simulink model "smm_with_grf_tilting_2d"  (R2014b)
settings: Solver=FixedStepDiscrete  StartTime=0.0  StopTime=inf  FixedStep=sample_time  RelTol=1e-3
undefined symbols (not defined in the file or in its folder): A_lpf_dtau, A_lpf_leg_spring, alpha_apex, alpha_max, alpha_min, B1_lpf_dtau, B1_lpf_leg_spring, B2_lpf_dtau, B2_lpf_leg_spring, boom_mount_angle, boom_pelvis_offset_angle, c_energy, contact_threshold, control_start_time, d_y_boom_com_offset, d_y_boom_hip_offset, d_y_com, desired_torso_angle, dx_avg_desired, enable_torso_wave, fcut_contact, ff_energy_l, ff_energy_r, g, g_reduced, h_boom, HIP_MTR_MAX_CONT_TORQUE, i_robot, initial_com_height, initial_dx, j_leg, j_motor, j_rotor, j_segments, k0_virtual, k_placement, k_sea, kd_lateral, kd_motor, kd_torso, kp_lateral, kp_motor, kp_raibert, kp_torso, l0_leg, l0_min_flight_time, l0_virtual, l0_virtual_raibert, l_boom_projected, l_max, l_retract_delta, l_retract_swing_max, l_retract_swing_min, l_seg, l_yaw_center_to_pelvis, lambda1, lambda2, lateral_offset, lateral_target_angle_left, lateral_target_angle_right ... (+40)
libraries: simulink x24, slrtlib x4, simulink_extras x2
(part 1 of 4)
settings Model: BufferReuse=off  Creator=wmartin  LastModifiedBy=wmartin
settings SolverCC: EnableConcurrentExecution=on
settings DataIOCC: MaxDataPoints=1000000000  SaveFormat=StructureWithTime
settings OptimizationCC: BlockReduction=off  OptimizeBlockIOStorage=off  BufferReuse=off  GlobalBufferReuse=off  ExpressionFolding=off  ExpressionDepthLimit=2147483647  LocalBlockOutputs=off  SimCompilerOptimization=On
settings DebuggingCC: UnderspecifiedInitializationDetection=Classic  MergeDetectMultiDrivingBlocksExec=none  StateNameClashWarn=warning
settings HardwareCC: ProdIntDivRoundTo=Zero  ProdEndianess=LittleEndian  ProdLongLongMode=on  ProdHWDeviceType=Generic->32-bit x86 compatible
settings ModelReferenceCC: UpdateModelReferenceTargets=IfOutOfDate  EnableParallelModelReferenceBuilds=on
settings RTWCC: SystemTargetFile=slrt.tlc  TemplateMakefile=slrt_default_tmf  Description=Simulink Real-Time  RTWVerbose=off  ProcessScript=slrt_make_rtw_hook  RTWCompilerOptimization=On
settings CodeAppCC: MaxIdLength=256
settings SimulinkRealTimeCC: GeneratePreprocessorConditionals=Disable all  EnableShiftOperators=on  RL32LogBufSizeModifier=100000000

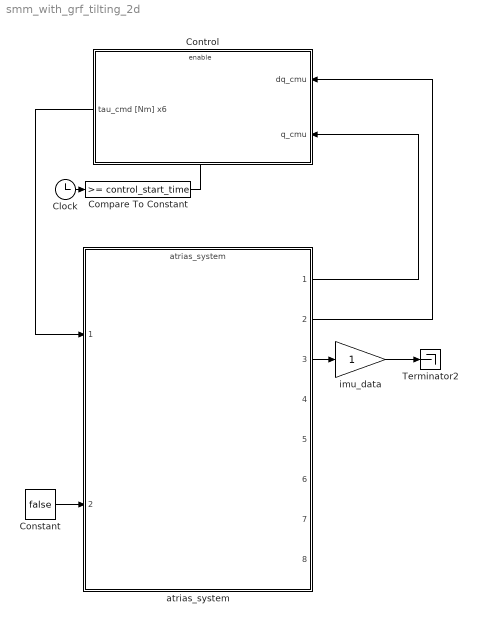
== system smm_with_grf_tilting_2d ==
  Clock : Clock
  Compare To Constant : simulink/Logic and Bit Operations/Compare To Constant  relop=>=  const=control_start_time  OutDataTypeStr=boolean
  Constant : Constant  Value=false
  Control : Subsystem
  Terminator2 : Terminator
  atrias_system : ModelReference  ModelNameDialog=atrias_system  SimulationMode=Normal  ModelReferenceVersion=1.2647  CopyOfModelName=atrias_system  DefaultDataLogging=on
  imu_data : Gain
  wires:
  Clock/1 -> Compare To Constant/1
  Compare To Constant/1 -> Control/Enable
  atrias_system/1 -> Control/2(q_cmu)
  atrias_system/2 -> Control/1(dq_cmu)
  Constant/1 -> atrias_system/2
  Control/1(tau_cmd [Nm] x6) -> atrias_system/1
  imu_data/1 -> Terminator2/1
  atrias_system/3 -> imu_data/1

== system smm_with_grf_tilting_2d/Control ==
  dq_cmu : Inport
  q_cmu : Inport  Port=2
  Enable : EnablePort  StatesWhenEnabling=reset
  Actuator Control : ModelReference  ModelNameDialog=actuator_control  SimulationMode=Normal  ModelReferenceVersion=1.66  CopyOfModelName=actuator_control  DefaultDataLogging=on
  Behavior Control : Subsystem
  tau_cmd [Nm] x6 : Outport  InitialOutput=[0 0 0 0 0 0]
  wires:
  q_cmu/1 -> Actuator Control/4, Behavior Control/2(q_cmu)
  dq_cmu/1 -> Actuator Control/5, Behavior Control/1(dq_cmu)
  Behavior Control/1(Motor Torque Command [Nm] x6) -> Actuator Control/1
  Actuator Control/1 -> tau_cmd [Nm] x6/1
  Behavior Control/2(SEA Torque Velocity Command [Nm] x4) -> Actuator Control/2
  Behavior Control/3(Force / Position Control [1/0] x4) -> Actuator Control/3

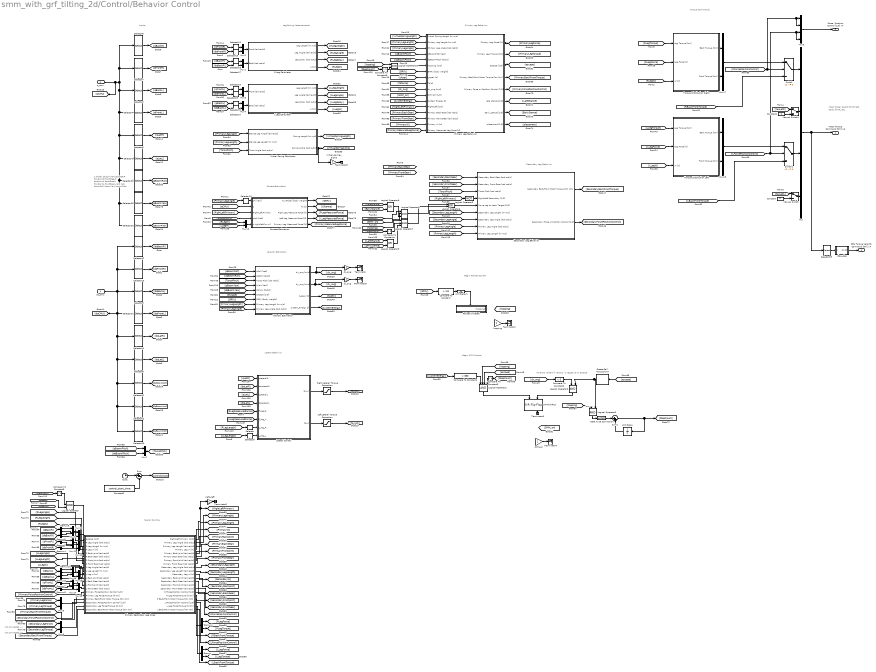
== system smm_with_grf_tilting_2d/Control/Behavior Control ==
  note: not connected -->
  note: Signal Routing
  note: Begin Raibert Control
  note: Begin SMM Control
  note: Velocity Estimation
  note: Contact Estimation
  note: Leg/Spring Measurements
  note: Lateral Behavior
  note: Torque Commands
  note: Secondary Leg Behavior
  note: Primary Leg Behavior
  note: Inputs
  note: q Order:
      |
      | backJointR
      | backGearR
      | frontJointR
      | frontGearR
      |
      | backJointL
      | backGearL
      | frontJointL
      | frontGearL
      |
      | latR
      | latL
      |
      | boomRoll
      | boomYaw
      | boomPitch
  note: Motor Order:
      |
      | backR
      | frontR
      | latR
      | backL
      | frontL
      | latL
  note: revert to raibert if velocity is negative on escape
  note: not connected -->
  dq_cmu : Inport
  q_cmu : Inport  Port=2
  Clock : Clock
  Compare To Constant : simulink/Logic and Bit Operations/Compare To Constant  relop=>  const=1.8  OutDataTypeStr=boolean
  Compare To Constant1 : simulink/Logic and Bit Operations/Compare To Constant  relop=>  const=350  OutDataTypeStr=boolean
  Compare To Constant2 : simulink/Logic and Bit Operations/Compare To Constant  relop=<  const=0  OutDataTypeStr=boolean  ZeroCross=off
  Compare To Constant3 : simulink/Logic and Bit Operations/Compare To Constant  relop=>  const=4  OutDataTypeStr=boolean
  Compare To Constant4 : simulink/Logic and Bit Operations/Compare To Constant  relop=>  const=2  OutDataTypeStr=boolean
  Compare To Constant5 : simulink/Logic and Bit Operations/Compare To Constant  relop=>  const=2  OutDataTypeStr=boolean
  Compare To Constant6 : simulink/Logic and Bit Operations/Compare To Constant  relop=>  const=2  OutDataTypeStr=boolean
  Constant : Constant  Value=0
  Constant1 : Constant  Value=0
  Constant2 : Constant  Value=control_start_time
  Contact Estimation : Subsystem
  Data Type Conversion : DataTypeConversion  OutDataTypeStr=uint32
  Demux{,1,3..10} (10 alike) : Demux  Outputs=2
  Detect Fall Nonpositive : simulink/Logic and Bit Operations/Detect Fall Nonpositive  vinit=0  InputProcessing=Inherited  OutDataTypeStr=boolean
  L Leg Calculator : Subsystem
  Lateral Control : MATLAB Function  TreatAsAtomicUnit=on
  Left Lateral Torque Saturation : Saturate  UpperLimit=max_torque_lateral  LowerLimit=-max_torque_lateral
      settings: AttributesFormatString=Top: %<UpperLimit>\nBottom: %<LowerLimit>
  Logical Operator{,2,5,10} (4 alike) : Logic  IconShape=distinctive  AllPortsSameDT=off  OutDataTypeStr=boolean
  Logical Operator1 : Logic  Inputs=4  IconShape=distinctive  AllPortsSameDT=off  OutDataTypeStr=boolean
  Logical Operator3 : Logic  Operator=NOT  AllPortsSameDT=off  OutDataTypeStr=boolean
  Logical Operator4 : Logic  Inputs=3  AllPortsSameDT=off  OutDataTypeStr=boolean
  Logical Operator6 : Logic  Operator=OR  AllPortsSameDT=off  OutDataTypeStr=boolean
  Logical Operator7 : Logic  Inputs=3  AllPortsSameDT=off  OutDataTypeStr=boolean
  Logical Operator8 : Logic  Operator=OR  AllPortsSameDT=off  OutDataTypeStr=boolean
  Logical Operator9 : Logic  Operator=OR  AllPortsSameDT=off  OutDataTypeStr=boolean
  Manual Switch : ManualSwitch
  Manual Switch1 : ManualSwitch
  Mux : Mux
  Mux{1..2,4..19} (18 alike) : Mux  Inputs=2
  Mux3 : Mux
  Primary Leg Behavior : Subsystem
  Primary Secondary Leg Swap : Subsystem
  R Leg Calculator : Subsystem
  Raibert Initiated : Subsystem
  Right Lateral Torque Saturation : Saturate  UpperLimit=max_torque_lateral  LowerLimit=-max_torque_lateral
      settings: AttributesFormatString=Top: %<UpperLimit>\nBottom: %<LowerLimit>
  S-R Flip-Flop : simulink_extras/Flip Flops/S-R Flip-Flop  initial_condition=0
  SMM_on : Gain
  Secondary Leg Behavior : Subsystem
  Selector{,3,14..17,19,24..27} (11 alike) : Selector  InputPortWidth=2  Indices=[1]
  Selector1 : Selector  InputPortWidth=13  Indices=[10]
  Selector10 : Selector  InputPortWidth=13  Indices=[7 8]
  Selector11 : Selector  InputPortWidth=13  Indices=[9]
  Selector12 : Selector  InputPortWidth=13  Indices=[1 2]
  Selector13 : Selector  InputPortWidth=13  Indices=[3 4]
  Selector18 : Selector  InputPortWidth=13  Indices=[13]
  Selector2 : Selector  InputPortWidth=13  Indices=[5 6]
  Selector20 : Selector  InputPortWidth=13  Indices=[13]
  Selector21 : Selector  InputPortWidth=13  Indices=[11]
  Selector22 : Selector  InputPortWidth=13  Indices=[12]
  Selector23 : Selector  InputPortWidth=13  Indices=[11]
  Selector28 : Selector  InputPortWidth=13  Indices=[12]
  Selector33 : Selector  InputPortWidth=6  Indices=[1 2 4 5]
  Selector4 : Selector  InputPortWidth=13  Indices=[7 8]
  Selector5 : Selector  InputPortWidth=13  Indices=[9]
  Selector6 : Selector  InputPortWidth=13  Indices=[1 2]
  Selector7 : Selector  InputPortWidth=13  Indices=[3 4]
  Selector8 : Selector  InputPortWidth=13  Indices=[10]
  Selector9 : Selector  InputPortWidth=13  Indices=[5 6]
  Sum : Sum  Inputs=|+-
  Sum1 : Sum  Inputs=|++  OutMin=0
  Switch : Switch  Criteria=u2 ~= 0
  Switch1 : Switch  Criteria=u2 ~= 0
  Terminator{,1..6} (7 alike) : Terminator
  Torque Distribution Left : Subsystem
  Torque Distribution Right : Subsystem
  Unit Delay : UnitDelay  SampleTime=-1
  Unit Delay1 : UnitDelay  SampleTime=sample_time
  Velocity Estimation : Subsystem
  Virtual Spring Calculator : Subsystem
  dtau_des : Subsystem
  dx_avg : Gain
  dy_avg : Gain
  hopping : Gain
  right_left : Gain
  virtual_spring_alpha : Gain
  Motor Torque Command [Nm] x6 : Outport  OutputWhenDisabled=reset  InitialOutput=[0 0 0 0 0 0]
  SEA Torque Velocity Command [Nm] x4 : Outport  Port=2  OutputWhenDisabled=reset  InitialOutput=[0 0 0 0 0 0]
  Force / Position Control [1/0] x4 : Outport  Port=3  OutputWhenDisabled=reset  InitialOutput=[0 0 0 0 0 0]
  wires:
  Unit Delay1/1 -> Raibert Initiated/Enable
  [escape] -> Logical Operator/2
  Logical Operator9/1 -> Logical Operator7/3
  Logical Operator8/1 -> Logical Operator4/3
  [SMM_on] -> Logical Operator4/2
  [hopping] -> Logical Operator4/1
  [LateStance] -> Logical Operator9/1
  [EarlyStance] -> Logical Operator9/2
  [LateStance] -> Logical Operator8/1
  [EarlyStance] -> Logical Operator8/2
  Primary Leg Behavior/7(early_stance [1/0]) -> [EarlyStance]
  Logical Operator6/1 -> Secondary Leg Behavior/5(Move Leg to Apex Target [1/0])
  Logical Operator7/1 -> Logical Operator6/2
  Compare To Constant4/1 -> Logical Operator7/2
  [hopping] -> Logical Operator7/1
  [StepCount] -> Compare To Constant4/1
  Compare To Constant3/1 -> Logical Operator1/4
  [StepCount] -> Compare To Constant3/1
  [hopping] -> Logical Operator5/1
  Data Type Conversion/1 -> Sum1/1
  Logical Operator5/1 -> Data Type Conversion/1
  Sum1/1 -> Unit Delay/1, [StepCount]
  Unit Delay/1 -> Sum1/2
  [hopping] -> Logical Operator1/2
  [escape] -> Detect Fall Nonpositive/1
  Logical Operator4/1 -> Logical Operator6/1
  [PrimaryW] -> Primary Leg Behavior/16(Primary w [m])
  Switch1/1 -> Mux/3
  [LBackFrontTorque] -> Switch1/3
  Mux18/1 -> Switch1/1
  [RBackFrontTorque] -> Switch/3
  Mux17/1 -> Switch/1
  Torque Distribution Left/2(Front Torque [Nm]) -> Mux18/2
  Torque Distribution Left/1(Back Torque [Nm]) -> Mux18/1
  Torque Distribution Right/1(Back Torque [Nm]) -> Mux17/1
  Torque Distribution Right/2(Front Torque [Nm]) -> Mux17/2
  Manual Switch/1 -> Mux/4
  Manual Switch1/1 -> Mux/2
  Switch/1 -> Mux/1
  [LForcePositionControl] -> Switch1/2, Mux3/3, Mux3/4
  [RForcePositionControl] -> Switch/2, Mux3/1, Mux3/2
  Primary Leg Behavior/6(late stance [1/0]) -> [LateStance]
  Secondary Leg Behavior/1(Secondary Back/Front Motor Torque [Nm Nm]) -> [SecondaryBackFrontTorque]
  Secondary Leg Behavior/2(Secondary Force or Position Control [1/0]) -> [SecondaryForcePositionControl]
  [SecondaryBackGear] -> Secondary Leg Behavior/1(Secondary Back Gear [rad rad/s])
  [SecondaryFrontGear] -> Secondary Leg Behavior/2(Secondary Front Gear [rad rad/s])
  Logical Operator3/1 -> Secondary Leg Behavior/4(Right/Left Secondary [1/0])
  [RightLeftPrimary] -> Logical Operator3/1
  Primary Leg Behavior/5(Primary Force or Position Control [1/0]) -> [PrimaryForcePositionControl]
  Primary Leg Behavior/4(Primary Back/Front Motor Torque [Nm Nm]) -> [PrimaryBackFrontTorque]
  [PrimaryFrontGear] -> Primary Leg Behavior/15(Primary Front Gear [rad rad/s])
  [PrimaryBackGear] -> Primary Leg Behavior/14(Primary Back Gear [rad rad/s])
  Primary Secondary Leg Swap/1(Right/Left Primary [1/0]) -> [RightLeftPrimary], right_left/1
  Logical Operator/1 -> Primary Secondary Leg Swap/1(escape [1/0])
  Primary Secondary Leg Swap/21(L Back/Front Motor Torque [Nm Nm]) -> [LBackFrontTorque]
  Primary Secondary Leg Swap/18(R Back/Front Motor Torque [Nm Nm]) -> [RBackFrontTorque]
  Primary Secondary Leg Swap/16(R Force/Position Control [1/0]) -> [RForcePositionControl]
  Primary Secondary Leg Swap/19(L Force/Position Control [1/0]) -> [LForcePositionControl]
  Primary Secondary Leg Swap/11(Secondary Leg w [m]) -> [SecondaryW]
  Primary Secondary Leg Swap/15(Secondary Front Gear [rad rad/s]) -> [SecondaryFrontGear]
  Primary Secondary Leg Swap/14(Secondary Front Joint [rad rad/s]) -> [SecondaryFrontJoint]
  Primary Secondary Leg Swap/13(Secondary Back Gear [rad rad/s]) -> [SecondaryBackGear]
  Primary Secondary Leg Swap/12(Secondary Back Joint [rad rad/s]) -> [SecondaryBackJoint]
  Primary Secondary Leg Swap/8(Primary Front Gear [rad rad/s]) -> [PrimaryFrontGear]
  Primary Secondary Leg Swap/7(Primary Front Joint [rad rad/s]) -> [PrimaryFrontJoint]
  Primary Secondary Leg Swap/6(Primary Back Gear [rad rad/s]) -> [PrimaryBackGear]
  Primary Secondary Leg Swap/5(Primary Back Joint [rad rad/s]) -> [PrimaryBackJoint]
  [SecondaryBackFrontTorque] -> Primary Secondary Leg Swap/21(Secondary Back/Front Motor Torque [Nm Nm])
  [PrimaryBackFrontTorque] -> Primary Secondary Leg Swap/18(Primary Back/Front Motor Torque [Nm Nm])
  [SecondaryForcePositionControl] -> Primary Secondary Leg Swap/19(Secondary Force/Position Control [1/0])
  [PrimaryForcePositionControl] -> Primary Secondary Leg Swap/16(Primary Force/Position Control [1/0])
  Demux9/2 -> Mux13/2
  Demux9/1 -> Mux16/2
  Demux10/2 -> Mux13/1
  Demux10/1 -> Mux16/1
  [qBackL] -> Demux10/1
  [dqBackL] -> Demux9/1
  Demux8/2 -> Mux15/2
  Demux8/1 -> Mux14/2
  Demux7/2 -> Mux15/1
  Demux7/1 -> Mux14/1
  Mux15/1 -> Primary Secondary Leg Swap/15(L Front Gear [rad rad/s])
  Mux14/1 -> Primary Secondary Leg Swap/14(L Front Joint [rad rad/s])
  Mux13/1 -> Primary Secondary Leg Swap/13(L Back Gear [rad rad/s])
  Mux16/1 -> Primary Secondary Leg Swap/12(L Back Joint [rad rad/s])
  [dqFrontL] -> Demux8/1
  [qFrontL] -> Demux7/1
  Demux5/2 -> Mux10/2
  Demux5/1 -> Mux9/2
  Demux6/2 -> Mux10/1
  Demux6/1 -> Mux9/1
  [qBackR] -> Demux6/1
  [dqBackR] -> Demux5/1
  Demux4/2 -> Mux12/2
  Demux4/1 -> Mux11/2
  Demux3/2 -> Mux12/1
  Demux3/1 -> Mux11/1
  Mux12/1 -> Primary Secondary Leg Swap/8(R Front Gear [rad rad/s])
  Mux11/1 -> Primary Secondary Leg Swap/7(R Front Joint [rad rad/s])
  Mux10/1 -> Primary Secondary Leg Swap/6(R Back Gear [rad rad/s])
  Mux9/1 -> Primary Secondary Leg Swap/5(R Back Joint [rad rad/s])
  [dqFrontR] -> Demux4/1
  [qFrontR] -> Demux3/1
  Demux1/2 -> [RLegTorque]
  Demux1/1 -> [RLegForce]
  Primary Secondary Leg Swap/17(R Leg Force/Torque [N Nm]) -> Demux1/1
  Demux/2 -> [LLegTorque]
  Demux/1 -> [LLegForce]
  Primary Secondary Leg Swap/20(L Leg Force/Torque [N Nm]) -> Demux/1
  Primary Secondary Leg Swap/9(Secondary Leg Angle [rad rad/s]) -> [SecondaryLegAngle]
  Primary Secondary Leg Swap/10(Secondary Leg Length [rad rad/s]) -> [SecondaryLegLength]
  [PrimaryLegForce] -> Mux8/1
  [PrimaryLegTorque] -> Mux8/2
  Mux8/1 -> Primary Secondary Leg Swap/17(Primary Leg Force/Torque [N Nm])
  Mux6/1 -> Primary Secondary Leg Swap/20(Secondary Leg Force/Torque [N Nm])
  [SecondaryLegTorque] -> Mux6/2
  [SecondaryLegForce] -> Mux6/1
  [LLegW] -> Primary Secondary Leg Swap/11(L Leg w [m])
  [LLegLength] -> Primary Secondary Leg Swap/10(L Leg Length [m m/s])
  [LLegAngle] -> Primary Secondary Leg Swap/9(L Leg Angle [rad rad/s])
  [RLegW] -> Primary Secondary Leg Swap/4(R Leg w [m])
  [RLegLength] -> Primary Secondary Leg Swap/3(R Leg Length [m m/s])
  [RLegAngle] -> Primary Secondary Leg Swap/2(R Leg Angle [rad rad/s])
  Primary Secondary Leg Swap/3(Primary Leg Length [rad rad/s]) -> [PrimaryLegLength]
  Primary Secondary Leg Swap/4(Primary Leg w [m]) -> [PrimaryW]
  Primary Secondary Leg Swap/2(Primary Leg Angle [rad rad/s]) -> [PrimaryLegAngle]
  Mux3/1 -> Force / Position Control [1/0] x4/1
  S-R Flip-Flop/2 -> Terminator6/1
  Logical Operator2/1 -> S-R Flip-Flop/2
  Compare To Constant2/1 -> Logical Operator2/1
  Detect Fall Nonpositive/1 -> Logical Operator5/2, Logical Operator2/2
  [dx_avg] -> Compare To Constant2/1
  virtual_spring_alpha/1 -> Terminator3/1
  [VirtualSpringLength] -> Primary Leg Behavior/1(Virtual Spring Length [m m/s])
  [TorsoPitch] -> Secondary Leg Behavior/3(Torso Pitch [rad rad/s])
  Mux7/1 -> [TorsoPitch]
  [dqBoomPitch] -> Mux7/2
  [qBoomPitch] -> Mux7/1
  Virtual Spring Calculator/2(Spring Alpha [rad rad/s]) -> [VirtualSpringAlpha], virtual_spring_alpha/1
  [TorsoPitch] -> Virtual Spring Calculator/3(Torso Angle [rad rad/s])
  Virtual Spring Calculator/1(Spring Length [m m/s]) -> [VirtualSpringLength]
  [PrimaryLegLength] -> Virtual Spring Calculator/2(Stance Leg Length [m m/s])
  [PrimaryLegAngle] -> Virtual Spring Calculator/1("Stance Leg Angle [rad rad/s] ")
  [RightLeftPrimary] -> Primary Leg Behavior/13(Right/Left [1/0])
  [escape] -> Logical Operator1/3
  Logical Operator1/1 -> S-R Flip-Flop/1
  [systemEnergy] -> Primary Leg Behavior/12(System Energy [J])
  [SMM_on] -> Primary Leg Behavior/11(SMM On [1/0])
  Compare To Constant1/1 -> Logical Operator1/1
  SMM_on/1 -> Terminator4/1
  ? -> SMM_on/1, [SMM_on]
  [systemEnergy] -> Compare To Constant1/1
  Velocity Estimation/4(system_energy [J]) -> [systemEnergy]
  [tStance] -> Primary Leg Behavior/9(Ts [s])
  [dx_avg] -> Primary Leg Behavior/10(dx_avg [m/s])
  dy_avg/1 -> Terminator5/1
  Velocity Estimation/3(t_apex [s]) -> [tApex]
  [tApex] -> Primary Leg Behavior/8(t_apex [s])
  Velocity Estimation/2(dy_avg [m/s]) -> [dy_avg], dy_avg/1
  Compare To Constant/1 -> Unit Delay1/1
  right_left/1 -> Terminator2/1
  [SecondaryLegLength] -> Secondary Leg Behavior/6(Secondary Leg Length [m m/s])
  [SecondaryLegAngle] -> Secondary Leg Behavior/7(Secondary Leg Angle [rad rad/s])
  [RightLeftPrimary] -> Contact Estimation/3(Right/Left Primary)
  [qCMU] -> Contact Estimation/2(q)
  [LLegW] -> Torque Distribution Left/3(w [m])
  [LLegForce] -> Torque Distribution Left/2(Leg Force [N])
  [LLegTorque] -> Torque Distribution Left/1(Leg Torque [Nm])
  hopping/1 -> Terminator1/1
  dx_avg/1 -> Terminator/1
  Velocity Estimation/1(dx_avg [m/s]) -> [dx_avg], dx_avg/1
  Primary Leg Behavior/2(Primary Leg Torque [Nm]) -> [PrimaryLegTorque]
  Primary Leg Behavior/1(Primary Leg Force [N]) -> [PrimaryLegForce]
  [PrimaryLegAngle] -> Primary Leg Behavior/3(Primary Leg Angle [rad rad/s])
  [dqBoomPitch] -> Primary Leg Behavior/5(dqBoomPitch [rad/s])
  [qBoomPitch] -> Primary Leg Behavior/4(qBoomPitch [rad])
  [GRFy] -> Primary Leg Behavior/7(GRFy [body weight])
  Logical Operator10/1 -> Primary Leg Behavior/6(hopping [1/0])
  [PrimaryLegLength] -> Primary Leg Behavior/2(Primary Leg Length [m m/s])
  Primary Leg Behavior/3(escape [1/0]) -> [escape]
  L Leg Calculator/4(w [m]) -> [LLegW]
  R Leg Calculator/4(w [m]) -> [RLegW]
  Selector26/1 -> Mux4/1
  Selector27/1 -> Mux4/2
  Selector25/1 -> Mux5/2
  Selector24/1 -> Mux5/1
  L Leg Calculator/3(Leg Splay [rad rad/s]) -> [LLegSplay]
  L Leg Calculator/2(Leg Angle [rad rad/s]) -> [LLegAngle]
  L Leg Calculator/1("Leg Length [m m/s] ") -> [LLegLength]
  Mux4/1 -> L Leg Calculator/2(Back [rad rad/s])
  Mux5/1 -> L Leg Calculator/1(Front [rad rad/s])
  [dqFrontL] -> Selector25/1
  [qFrontL] -> Selector24/1
  [dqBackL] -> Selector27/1
  [qBackL] -> Selector26/1
  Selector23/1 -> [qBoomRoll]
  Selector21/1 -> [dqBoomRoll]
  dq_cmu/1 -> Selector9/1, Selector13/1, Selector12/1, [dqCMU], Selector10/1, Selector11/1, Selector8/1, Selector21/1, Selector22/1, Selector20/1
  ? -> [hopping], hopping/1
  [GRFy] -> Compare To Constant/1
  Contact Estimation/2(Ts [s]) -> [tStance]
  Selector22/1 -> [dqBoomYaw]
  [RLegTorque] -> Torque Distribution Right/1(Leg Torque [Nm])
  [RLegForce] -> Torque Distribution Right/2(Leg Force [N])
  Selector20/1 -> [dqBoomPitch]
  Contact Estimation/1(F_vertical [body weight]) -> [GRFy]
  Selector19/1 -> Contact Estimation/1(phi [rad])
  [PrimaryLegAngle] -> Selector19/1
  [qBoomPitch] -> Contact Estimation/4(pitch [rad])
  Selector18/1 -> [qBoomPitch]
  q_cmu/1 -> [qCMU], Selector1/1, Selector23/1, Selector28/1, Selector18/1, Selector5/1, Selector4/1, Selector2/1, Selector7/1, Selector6/1
  Mux19/1 -> Contact Estimation/5(w right/left [m m])
  Selector16/1 -> Mux1/1
  Selector17/1 -> Mux1/2
  Selector15/1 -> Mux2/2
  Selector14/1 -> Mux2/1
  [RLegW] -> Torque Distribution Right/3(w [m])
  [tauLatL] -> Manual Switch/1
  [tauLatR] -> Manual Switch1/1
  R Leg Calculator/3(Leg Splay [rad rad/s]) -> [RLegSplay]
  R Leg Calculator/2(Leg Angle [rad rad/s]) -> [RLegAngle]
  R Leg Calculator/1("Leg Length [m m/s] ") -> [RLegLength]
  Mux1/1 -> R Leg Calculator/2(Back [rad rad/s])
  Mux2/1 -> R Leg Calculator/1(Front [rad rad/s])
  [dqFrontR] -> Selector15/1
  [qFrontR] -> Selector14/1
  [dqBackR] -> Selector17/1
  [qBackR] -> Selector16/1
  Selector10/1 -> [dqFrontL]
  Selector9/1 -> [dqBackL]
  Selector13/1 -> [dqFrontR]
  Selector12/1 -> [dqBackR]
  Selector11/1 -> [dqLatR]
  Selector8/1 -> [dqLatL]
  Constant/1 -> Manual Switch/2
  Constant1/1 -> Manual Switch1/2
  Clock/1 -> Sum/1
  Constant2/1 -> Sum/2
  Selector5/1 -> [qLatR]
  Selector1/1 -> [qLatL]
  Selector6/1 -> [qBackR]
  Selector7/1 -> [qFrontR]
  Selector2/1 -> [qBackL]
  Selector4/1 -> [qFrontL]
  Sum/1 -> [controlClock]
  Lateral Control/1(tau_r) -> Right Lateral Torque Saturation/1
  Lateral Control/2(tau_l) -> Left Lateral Torque Saturation/1
  Right Lateral Torque Saturation/1 -> [tauLatR]
  Left Lateral Torque Saturation/1 -> [tauLatL]
  Primary Leg Behavior/8(placement [1/0]) -> [placement]
  Contact Estimation/3(Right Leg Measure Force [N]) -> [RLegMeasuredForce]
  [StepCount] -> Compare To Constant5/1
  Compare To Constant5/1 -> Logical Operator/1
  [PrimaryLegAngle] -> Secondary Leg Behavior/8(Primary Leg Angle [rad rad/s])
  Selector33/1 -> dtau_des/1(x)
  dtau_des/1(dx/dt) -> SEA Torque Velocity Command [Nm] x4/1
  Mux/1 -> Selector33/1, Motor Torque Command [Nm] x6/1
  [dqLatR] -> Lateral Control/2(dqLateralR)
  [qLatR] -> Lateral Control/1(qLateralR)
  [dqLatL] -> Lateral Control/4(dqLateralL)
  [qLatL] -> Lateral Control/3(qLateralL)
  [RLegLength] -> Selector/1
  [LLegLength] -> Selector3/1
  [RLegMeasuredForce] -> Lateral Control/5(F_leg_R)
  [LLegMeasuredForce] -> Lateral Control/6(F_leg_L)
  [RLegW] -> Mux19/1
  [LLegW] -> Mux19/2
  Contact Estimation/4(Left Leg Measure Force [N]) -> [LLegMeasuredForce]
  [PrimaryLegLength] -> Secondary Leg Behavior/9(Primary Leg Length [m m/s])
  Selector/1 -> Lateral Control/7(L_leg_R)
  Selector3/1 -> Lateral Control/8(L_leg_L)
  [PrimaryMeasuredLegForce] -> Primary Leg Behavior/17(Primary Measured Leg Force [N])
  Contact Estimation/5(Primary Leg Measured Force [N]) -> [PrimaryMeasuredLegForce]
  [StepCount] -> Compare To Constant6/1
  Compare To Constant6/1 -> Logical Operator10/2
  [hopping] -> Logical Operator10/1
  [qBoomRoll] -> Velocity Estimation/1(qRoll [rad])
  [dqBoomRoll] -> Velocity Estimation/2(dqRoll [rad/s])
  [TorsoPitch] -> Velocity Estimation/3(Torso Pitch [rad rad/s])
  [qBoomYaw] -> Velocity Estimation/4(qYaw [rad])
  [dqBoomYaw] -> Velocity Estimation/5(dqYaw [rad/s])
  [GRFy] -> Velocity Estimation/7(GRFy [body weight])
  [escape] -> Velocity Estimation/6(escape [1/0])
  [PrimaryLegLength] -> Velocity Estimation/8(Primary Leg Length [m m/s])
  [PrimaryLegAngle] -> Velocity Estimation/9(Primary Leg Angle [rad rad/s])
  Selector28/1 -> [qBoomYaw]

== system smm_with_grf_tilting_2d/Control/Behavior Control/Contact Estimation ==
  phi [rad] : Inport
  q : Inport  Port=2
  Right/Left Primary : Inport  Port=3
  pitch [rad] : Inport  Port=4
  w right/left [m m] : Inport  Port=5
  Compare To Constant : simulink/Logic and Bit Operations/Compare To Constant  relop=>=  const=loaded_threshold  OutDataTypeStr=boolean
  Compare To Constant1 : simulink/Logic and Bit Operations/Compare To Constant  relop=>=  const=0.040  OutDataTypeStr=boolean
  Constant : Constant  Value=m_total_real*g
  Contact Time : Subsystem
  Detect Decrease : simulink/Logic and Bit Operations/Detect Decrease  vinit=0.0  InputProcessing=Inherited  OutDataTypeStr=boolean
  Divide : Product  Inputs=*/
  Last Contact Time : Subsystem
  Leg Force Measurements : Subsystem
  Logical Operator : Logic  AllPortsSameDT=off  OutDataTypeStr=boolean
  Switch1 : Switch  Criteria=u2 ~= 0
  Vertical Spring Force : Subsystem
  two_pole_filter : DiscreteTransferFcn  Numerator=[(1-2*exp(-fcut_contact*sample_time)+exp(-2*fcut_contact*sample_time)) 0 0]  Denominator=[1 (-2*exp(-fcut_contact*sample_time)) (exp(-2*fcut_contact*sample_time))]  SampleTime=sample_time
  F_vertical [body weight] : Outport
  Ts [s] : Outport  Port=2
  Right Leg Measure Force [N] : Outport  Port=3
  Left Leg Measure Force [N] : Outport  Port=4
  Primary Leg Measured Force [N] : Outport  Port=5
  wires:
  Divide/1 -> Compare To Constant/1, F_vertical [body weight]/1
  Compare To Constant1/1 -> Logical Operator/2
  Detect Decrease/1 -> Logical Operator/1
  Logical Operator/1 -> Last Contact Time/Trigger
  Compare To Constant/1 -> Contact Time/Enable, Detect Decrease/1
  Contact Time/1(ts [s]) -> Compare To Constant1/1, Last Contact Time/1(ts [s])
  Last Contact Time/1(Ts [s]) -> Ts [s]/1
  phi [rad]/1 -> Vertical Spring Force/2(phi [rad])
  w right/left [m m]/1 -> Leg Force Measurements/2(w right/left [m m])
  pitch [rad]/1 -> Vertical Spring Force/1(theta [rad])
  Leg Force Measurements/2(Left Leg Force [N]) -> Left Leg Measure Force [N]/1, Switch1/3
  Leg Force Measurements/1(Right Leg Force [N]) -> Right Leg Measure Force [N]/1, Switch1/1
  q/1 -> Leg Force Measurements/1(q)
  two_pole_filter/1 -> Divide/1
  Constant/1 -> Divide/2
  Vertical Spring Force/1(Vertical Force [N]) -> two_pole_filter/1
  Switch1/1 -> Primary Leg Measured Force [N]/1, Vertical Spring Force/3(Force [N])
  Right/Left Primary/1 -> Switch1/2

== system smm_with_grf_tilting_2d/Control/Behavior Control/L Leg Calculator ==
  Front [rad rad/s] : Inport
  Back [rad rad/s] : Inport  Port=2
  Demux1 : Demux  Outputs=2
  Gain1 : Gain  Gain=2*l_seg
  Gain2 : Gain  Gain=l_seg
  Gain3 : Gain  Gain=-1
  Gain4 : Gain  Gain=0.5
  Gain5 : Gain  Gain=0.5
  Gain6 : Gain  Gain=2
  Mux1 : Mux  Inputs=2
  Product : Product  RndMeth=Zero
  Sum4 : Sum  Inputs=+|+
  Sum5 : Sum  Inputs=+|-
  Trigonometric Function : Trigonometry  Operator=cos
  Trigonometric Function1 : Trigonometry
  "Leg Length [m m/s] " : Outport
  Leg Angle [rad rad/s] : Outport  Port=2
  Leg Splay [rad rad/s] : Outport  Port=3
  w [m] : Outport  Port=4
  wires:
  Gain6/1 -> w [m]/1
  Gain4/1 -> Trigonometric Function1/1, Trigonometric Function/1
  Trigonometric Function/1 -> Gain1/1
  Gain1/1 -> Mux1/1
  Trigonometric Function1/1 -> Gain2/1
  Product/1 -> Mux1/2
  Front [rad rad/s]/1 -> Sum5/2, Sum4/2
  Back [rad rad/s]/1 -> Sum4/1, Sum5/1
  Demux1/2 -> Gain3/1
  Gain3/1 -> Product/2
  Demux1/1 -> Gain4/1
  Gain2/1 -> Product/1, Gain6/1
  Sum5/1 -> Leg Splay [rad rad/s]/1, Demux1/1
  Mux1/1 -> "Leg Length [m m/s] "/1
  Sum4/1 -> Gain5/1
  Gain5/1 -> Leg Angle [rad rad/s]/1

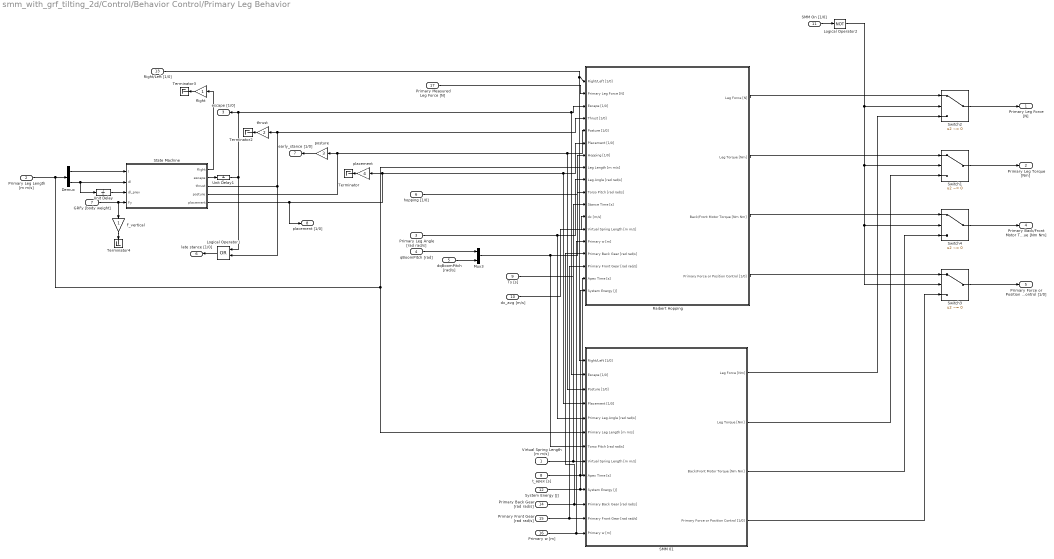
== system smm_with_grf_tilting_2d/Control/Behavior Control/Primary Leg Behavior ==
  Virtual Spring Length [m m/s] : Inport
  Primary Leg Length [m m/s] : Inport  Port=2
  Primary Leg Angle [rad rad/s] : Inport  Port=3
  qBoomPitch [rad] : Inport  Port=4
  dqBoomPitch [rad/s] : Inport  Port=5
  hopping [1/0] : Inport  Port=6
  GRFy [body weight] : Inport  Port=7
  t_apex [s] : Inport  Port=8
  Ts [s] : Inport  Port=9
  dx_avg [m/s] : Inport  Port=10
  SMM On [1/0] : Inport  Port=11
  System Energy [J] : Inport  Port=12
  Right/Left [1/0] : Inport  Port=13
  Primary Back Gear [rad rad/s] : Inport  Port=14
  Primary Front Gear [rad rad/s] : Inport  Port=15
  Primary w [m] : Inport  Port=16
  Primary Measured Leg Force [N] : Inport  Port=17
  Demux : Demux  Outputs=2
  F_vertical : Gain
  Logical Operator1 : Logic  Operator=OR  AllPortsSameDT=off  OutDataTypeStr=boolean
  Logical Operator2 : Logic  Operator=NOT  AllPortsSameDT=off  OutDataTypeStr=boolean
  Mux3 : Mux  Inputs=2
  Raibert Hopping : Subsystem
  SMM 01 : Subsystem
  State Machine : State Transition Table  TreatAsAtomicUnit=on
  Switch{1..4} (4 alike) : Switch  Criteria=u2 ~= 0
  Terminator{,2..4} (4 alike) : Terminator
  Unit Delay : UnitDelay  SampleTime=-1
  Unit Delay1 : UnitDelay  SampleTime=sample_time
  flight : Gain
  placement : Gain  Gain=4
  posture : Gain  Gain=3
  thrust : Gain  Gain=2
  Primary Leg Force [N] : Outport
  Primary Leg Torque [Nm] : Outport  Port=2
  escape [1/0] : Outport  Port=3
  Primary Back/Front Motor Torque [Nm Nm] : Outport  Port=4
  Primary Force or Position Control [1/0] : Outport  Port=5
  late stance [1/0] : Outport  Port=6
  early_stance [1/0] : Outport  Port=7
  placement [1/0] : Outport  Port=8
  wires:
  Unit Delay1/1 -> Logical Operator1/1, escape [1/0]/1, Raibert Hopping/3(Escape [1/0]), SMM 01/2(Escape [1/0])
  State Machine/2(escape) -> Unit Delay1/1
  Switch3/1 -> Primary Force or Position Control [1/0]/1
  Logical Operator1/1 -> late stance [1/0]/1
  Primary Leg Angle [rad rad/s]/1 -> Raibert Hopping/9(Leg Angle [rad rad/s]), SMM 01/5(Primary Leg Angle [rad rad/s])
  Primary Back Gear [rad rad/s]/1 -> Raibert Hopping/15(Primary Back Gear [rad rad/s]), SMM 01/11(Primary Back Gear [rad rad/s])
  Virtual Spring Length [m m/s]/1 -> Raibert Hopping/13(Virtual Spring Length [m m/s]), SMM 01/8(Virtual Spring Length [m m/s])
  Right/Left [1/0]/1 -> Raibert Hopping/1(Right/Left [1/0]), SMM 01/1(Right/Left [1/0])
  System Energy [J]/1 -> Raibert Hopping/18(System Energy [J]), SMM 01/10(System Energy [J])
  t_apex [s]/1 -> Raibert Hopping/17(Apex Time [s]), SMM 01/9(Apex Time [s])
  Switch1/1 -> Primary Leg Torque [Nm]/1
  Switch2/1 -> Primary Leg Force [N]/1
  dx_avg [m/s]/1 -> Raibert Hopping/12(dx [m/s])
  Ts [s]/1 -> Raibert Hopping/11(Stance Time [s])
  hopping [1/0]/1 -> Raibert Hopping/7(Hopping [1/0])
  Demux/1 -> State Machine/1(l)
  flight/1 -> Terminator3/1
  F_vertical/1 -> Terminator4/1
  Primary Leg Length [m m/s]/1 -> Demux/1, Raibert Hopping/8(Leg Length [m m/s]), SMM 01/6(Primary Leg Length [m m/s])
  thrust/1 -> Terminator2/1
  posture/1 -> early_stance [1/0]/1
  placement/1 -> Terminator/1
  State Machine/1(flight) -> flight/1
  State Machine/3(thrust) -> thrust/1, Raibert Hopping/4(Thrust [1/0]), Logical Operator1/2
  Demux/2 -> State Machine/2(dl), Unit Delay/1
  GRFy [body weight]/1 -> State Machine/4(Fy), F_vertical/1
  Unit Delay/1 -> State Machine/3(dl_prev)
  dqBoomPitch [rad/s]/1 -> Mux3/2
  qBoomPitch [rad]/1 -> Mux3/1
  Mux3/1 -> Raibert Hopping/10(Torso Pitch [rad rad/s]), SMM 01/7(Torso Pitch [rad rad/s])
  State Machine/4(posture) -> Raibert Hopping/5(Posture [1/0]), SMM 01/3(Posture [1/0]), posture/1
  State Machine/5(placement) -> placement [1/0]/1, placement/1, SMM 01/4(Placement [1/0]), Raibert Hopping/6(Placement [1/0])
  Primary w [m]/1 -> SMM 01/13(Primary w [m]), Raibert Hopping/14(Primary w [m])
  Switch4/1 -> Primary Back/Front Motor Torque [Nm Nm]/1
  SMM On [1/0]/1 -> Logical Operator2/1
  Logical Operator2/1 -> Switch2/2, Switch1/2, Switch4/2, Switch3/2
  Raibert Hopping/1(Leg Force [N]) -> Switch2/1
  Raibert Hopping/2(Leg Torque [Nm]) -> Switch1/1
  Raibert Hopping/3(Back/Front Motor Torque [Nm Nm]) -> Switch4/1
  Raibert Hopping/4(Primary Force or Position Control [1/0]) -> Switch3/1
  SMM 01/4(Primary Force or Position Control [1/0]) -> Switch3/3
  SMM 01/1(Leg Force [Nm]) -> Switch2/3
  SMM 01/2(Leg Torque [Nm]) -> Switch1/3
  SMM 01/3(Back/Front Motor Torque [Nm Nm]) -> Switch4/3
  Primary Front Gear [rad rad/s]/1 -> Raibert Hopping/16(Primary Front Gear [rad rad/s]), SMM 01/12(Primary Front Gear [rad rad/s])
  Primary Measured Leg Force [N]/1 -> Raibert Hopping/2(Primary Leg Force [N])

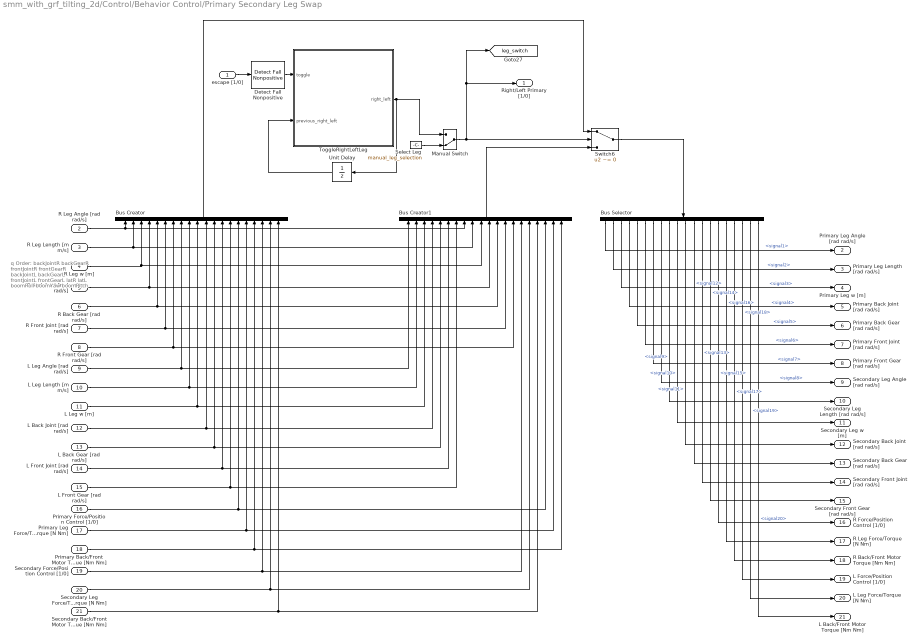
== system smm_with_grf_tilting_2d/Control/Behavior Control/Primary Secondary Leg Swap ==
  note: q Order:
      |
      | backJointR
      | backGearR
      | frontJointR
      | frontGearR
      |
      | backJointL
      | backGearL
      | frontJointL
      | frontGearL
      |
      | latR
      | latL
      |
      | boomRoll
      | boomYaw
      | boomPitch
  escape [1/0] : Inport
  R Leg Angle [rad rad/s] : Inport  Port=2
  R Leg Length [m m/s] : Inport  Port=3
  R Leg w [m] : Inport  Port=4
  R Back Joint [rad rad/s] : Inport  Port=5
  R Back Gear [rad rad/s] : Inport  Port=6
  R Front Joint [rad rad/s] : Inport  Port=7
  R Front Gear [rad rad/s] : Inport  Port=8
  L Leg Angle [rad rad/s] : Inport  Port=9
  L Leg Length [m m/s] : Inport  Port=10
  L Leg w [m] : Inport  Port=11
  L Back Joint [rad rad/s] : Inport  Port=12
  L Back Gear [rad rad/s] : Inport  Port=13
  L Front Joint [rad rad/s] : Inport  Port=14
  L Front Gear [rad rad/s] : Inport  Port=15
  Primary Force/Position Control [1/0] : Inport  Port=16
  Primary Leg Force/Torque [N Nm] : Inport  Port=17
  Primary Back/Front Motor Torque [Nm Nm] : Inport  Port=18
  Secondary Force/Position Control [1/0] : Inport  Port=19
  Secondary Leg Force/Torque [N Nm] : Inport  Port=20
  Secondary Back/Front Motor Torque [Nm Nm] : Inport  Port=21
  Bus Creator : BusCreator  Inputs=20
  Bus Creator1 : BusCreator  Inputs=20
  Bus Selector : BusSelector  OutputSignals=signal1,signal2,signal3,signal4,signal5,signal6,signal7,signal8,signal9,signal10,signal11,signal12,signal13,signal14,signal15,signal16,signal17,signal18,signal19,signal20
  Detect Fall Nonpositive : simulink/Logic and Bit Operations/Detect Fall Nonpositive  vinit=0  InputProcessing=Inherited  OutDataTypeStr=boolean
  Manual Switch : ManualSwitch  CurrentSetting=0
  Select Leg : Constant  Value=manual_leg_selection  OutDataTypeStr=boolean
  Switch6 : Switch  Criteria=u2 ~= 0  OutDataTypeStr=Inherit: Inherit via back propagation  ZeroCross=off
  ToggleRightLeftLeg : MATLAB Function  TreatAsAtomicUnit=on
      settings: MinAlgLoopOccurrences=on
  Unit Delay : UnitDelay  SampleTime=sample_time
  Right/Left Primary [1/0] : Outport
  Primary Leg Angle [rad rad/s] : Outport  Port=2
  Primary Leg Length [rad rad/s] : Outport  Port=3
  Primary Leg w [m] : Outport  Port=4
  Primary Back Joint [rad rad/s] : Outport  Port=5
  Primary Back Gear [rad rad/s] : Outport  Port=6
  Primary Front Joint [rad rad/s] : Outport  Port=7
  Primary Front Gear [rad rad/s] : Outport  Port=8
  Secondary Leg Angle [rad rad/s] : Outport  Port=9
  Secondary Leg Length [rad rad/s] : Outport  Port=10
  Secondary Leg w [m] : Outport  Port=11
  Secondary Back Joint [rad rad/s] : Outport  Port=12
  Secondary Back Gear [rad rad/s] : Outport  Port=13
  Secondary Front Joint [rad rad/s] : Outport  Port=14
  Secondary Front Gear [rad rad/s] : Outport  Port=15
  R Force/Position Control [1/0] : Outport  Port=16
  R Leg Force/Torque [N Nm] : Outport  Port=17
  R Back/Front Motor Torque [Nm Nm] : Outport  Port=18
  L Force/Position Control [1/0] : Outport  Port=19
  L Leg Force/Torque [N Nm] : Outport  Port=20
  L Back/Front Motor Torque [Nm Nm] : Outport  Port=21
  tag scope: leg_switch=global
  wires:
  Unit Delay/1 -> ToggleRightLeftLeg/2(previous_right_left)
  Detect Fall Nonpositive/1 -> ToggleRightLeftLeg/1(toggle)
  escape [1/0]/1 -> Detect Fall Nonpositive/1
  ToggleRightLeftLeg/1(right_left) -> Unit Delay/1, Manual Switch/1
  Manual Switch/1 -> [leg_switch], Right/Left Primary [1/0]/1, Switch6/2
  Select Leg/1 -> Manual Switch/2
  R Leg w [m]/1 -> Bus Creator1/10, Bus Creator/3
  R Leg Angle [rad rad/s]/1 -> Bus Creator1/8, Bus Creator/1
  R Leg Length [m m/s]/1 -> Bus Creator1/9, Bus Creator/2
  Bus Creator/1 -> Switch6/1
  Bus Creator1/1 -> Switch6/3
  R Back Joint [rad rad/s]/1 -> Bus Creator1/11, Bus Creator/4
  R Back Gear [rad rad/s]/1 -> Bus Creator1/12, Bus Creator/5
  R Front Joint [rad rad/s]/1 -> Bus Creator1/13, Bus Creator/6
  R Front Gear [rad rad/s]/1 -> Bus Creator1/14, Bus Creator/7
  L Leg Angle [rad rad/s]/1 -> Bus Creator1/1, Bus Creator/8
  L Leg Length [m m/s]/1 -> Bus Creator1/2, Bus Creator/9
  L Leg w [m]/1 -> Bus Creator1/3, Bus Creator/10
  L Back Joint [rad rad/s]/1 -> Bus Creator1/4, Bus Creator/11
  L Back Gear [rad rad/s]/1 -> Bus Creator1/5, Bus Creator/12
  L Front Joint [rad rad/s]/1 -> Bus Creator/13, Bus Creator1/6
  L Front Gear [rad rad/s]/1 -> Bus Creator1/7, Bus Creator/14
  Primary Force/Position Control [1/0]/1 -> Bus Creator1/18, Bus Creator/15
  Primary Leg Force/Torque [N Nm]/1 -> Bus Creator1/19, Bus Creator/16
  Primary Back/Front Motor Torque [Nm Nm]/1 -> Bus Creator1/20, Bus Creator/17
  Secondary Force/Position Control [1/0]/1 -> Bus Creator1/15, Bus Creator/18
  Secondary Leg Force/Torque [N Nm]/1 -> Bus Creator1/16, Bus Creator/19
  Secondary Back/Front Motor Torque [Nm Nm]/1 -> Bus Creator1/17, Bus Creator/20
  Switch6/1 -> Bus Selector/1
  Bus Selector/1 -> Primary Leg Angle [rad rad/s]/1  "<signal1>"
  Bus Selector/2 -> Primary Leg Length [rad rad/s]/1  "<signal2>"
  Bus Selector/3 -> Primary Leg w [m]/1  "<signal3>"
  Bus Selector/4 -> Primary Back Joint [rad rad/s]/1  "<signal4>"
  Bus Selector/5 -> Primary Back Gear [rad rad/s]/1  "<signal5>"
  Bus Selector/6 -> Primary Front Joint [rad rad/s]/1  "<signal6>"
  Bus Selector/7 -> Primary Front Gear [rad rad/s]/1  "<signal7>"
  Bus Selector/8 -> Secondary Leg Angle [rad rad/s]/1  "<signal8>"
  Bus Selector/9 -> Secondary Leg Length [rad rad/s]/1  "<signal9>"
  Bus Selector/10 -> Secondary Leg w [m]/1  "<signal10>"
  Bus Selector/11 -> Secondary Back Joint [rad rad/s]/1  "<signal11>"
  Bus Selector/12 -> Secondary Back Gear [rad rad/s]/1  "<signal12>"
  Bus Selector/13 -> Secondary Front Joint [rad rad/s]/1  "<signal13>"
  Bus Selector/14 -> Secondary Front Gear [rad rad/s]/1  "<signal14>"
  Bus Selector/15 -> R Force/Position Control [1/0]/1  "<signal15>"
  Bus Selector/16 -> R Leg Force/Torque [N Nm]/1  "<signal16>"
  Bus Selector/17 -> R Back/Front Motor Torque [Nm Nm]/1  "<signal17>"
  Bus Selector/18 -> L Force/Position Control [1/0]/1  "<signal18>"
  Bus Selector/19 -> L Leg Force/Torque [N Nm]/1  "<signal19>"
  Bus Selector/20 -> L Back/Front Motor Torque [Nm Nm]/1  "<signal20>"

== system smm_with_grf_tilting_2d/Control/Behavior Control/R Leg Calculator ==
  Front [rad rad/s] : Inport
  Back [rad rad/s] : Inport  Port=2
  Demux1 : Demux  Outputs=2
  Gain1 : Gain  Gain=2*l_seg
  Gain2 : Gain  Gain=l_seg
  Gain3 : Gain  Gain=-1
  Gain4 : Gain  Gain=0.5
  Gain5 : Gain  Gain=0.5
  Gain6 : Gain  Gain=2
  Mux1 : Mux  Inputs=2
  Product : Product  RndMeth=Zero
  Sum4 : Sum  Inputs=+|+
  Sum5 : Sum  Inputs=+|-
  Trigonometric Function : Trigonometry  Operator=cos
  Trigonometric Function1 : Trigonometry
  "Leg Length [m m/s] " : Outport
  Leg Angle [rad rad/s] : Outport  Port=2
  Leg Splay [rad rad/s] : Outport  Port=3
  w [m] : Outport  Port=4
  wires:
  Gain5/1 -> Leg Angle [rad rad/s]/1
  Sum4/1 -> Gain5/1
  Mux1/1 -> "Leg Length [m m/s] "/1
  Sum5/1 -> Demux1/1, Leg Splay [rad rad/s]/1
  Gain2/1 -> Gain6/1, Product/1
  Demux1/1 -> Gain4/1
  Gain3/1 -> Product/2
  Demux1/2 -> Gain3/1
  Back [rad rad/s]/1 -> Sum5/1, Sum4/1
  Front [rad rad/s]/1 -> Sum4/2, Sum5/2
  Product/1 -> Mux1/2
  Trigonometric Function1/1 -> Gain2/1
  Gain1/1 -> Mux1/1
  Trigonometric Function/1 -> Gain1/1
  Gain4/1 -> Trigonometric Function/1, Trigonometric Function1/1
  Gain6/1 -> w [m]/1

== system smm_with_grf_tilting_2d/Control/Behavior Control/Raibert Initiated ==
  Enable : EnablePort  StatesWhenEnabling=reset
  Constant : Constant
  Hopping? : Outport  InitialOutput=[0]
  wires:
  Constant/1 -> Hopping?/1

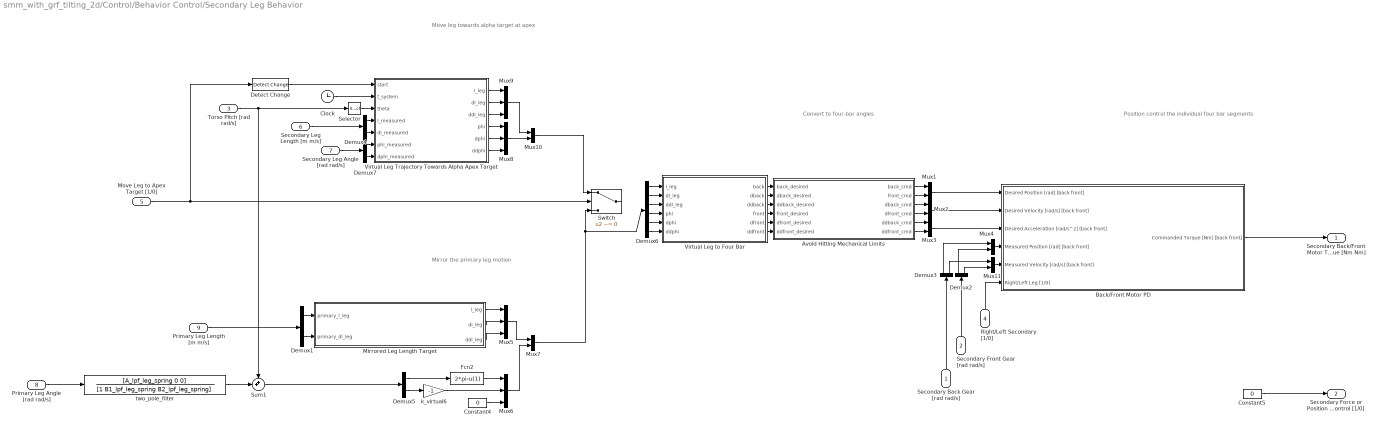
== system smm_with_grf_tilting_2d/Control/Behavior Control/Secondary Leg Behavior ==
  note: Mirror the primary
      | leg motion
  note: Move leg towards
      | alpha target at apex
  note: Position control the
      | individual four bar segments
  note: Convert to
      | four-bar angles
  Secondary Back Gear [rad rad/s] : Inport
  Secondary Front Gear [rad rad/s] : Inport  Port=2
  Torso Pitch [rad rad/s] : Inport  Port=3
  Right/Left Secondary [1/0] : Inport  Port=4
  Move Leg to Apex Target [1/0] : Inport  Port=5
  Secondary Leg Length [m m/s] : Inport  Port=6
  Secondary Leg Angle [rad rad/s] : Inport  Port=7
  Primary Leg Angle [rad rad/s] : Inport  Port=8
  Primary Leg Length [m m/s] : Inport  Port=9
  Avoid Hitting Mechanical Limits : MATLAB Function  TreatAsAtomicUnit=on
  Back/Front Motor PD : Subsystem
  Clock : Clock
  Constant4 : Constant  Value=0
  Constant5 : Constant  Value=0  OutDataTypeStr=boolean
  Demux{1..5,7} (6 alike) : Demux  Outputs=2
  Demux6 : Demux  Outputs=6
  Detect Change : simulink/Logic and Bit Operations/Detect Change  vinit=0  InputProcessing=Inherited  OutDataTypeStr=boolean
  Fcn2 : Fcn  Expr=2*pi-u(1)
  Mirrored Leg Length Target : MATLAB Function  TreatAsAtomicUnit=on
  Mux{1..4,7,10..11} (7 alike) : Mux  Inputs=2
  Mux{5..6,8..9} (4 alike) : Mux  Inputs=3
  Selector : Selector  InputPortWidth=2  Indices=[1]
  Sum1 : Sum  Inputs=++|
  Switch : Switch  Criteria=u2 ~= 0
  Virtual Leg Trajectory Towards Alpha Apex Target : MATLAB Function  TreatAsAtomicUnit=on
  Virtual Leg to Four Bar : MATLAB Function  TreatAsAtomicUnit=on
  k_virtual6 : Gain  Gain=-1
  two_pole_filter : DiscreteTransferFcn  Numerator=[A_lpf_leg_spring 0 0]  Denominator=[1 B1_lpf_leg_spring B2_lpf_leg_spring]  SampleTime=sample_time
  Secondary Back/Front Motor Torque [Nm Nm] : Outport
  Secondary Force or Position Control [1/0] : Outport  Port=2
  wires:
  Constant5/1 -> Secondary Force or Position Control [1/0]/1
  Back/Front Motor PD/1(Commanded Torque [Nm] [back front]) -> Secondary Back/Front Motor Torque [Nm Nm]/1
  Demux5/2 -> k_virtual6/1
  Demux5/1 -> Fcn2/1
  Primary Leg Angle [rad rad/s]/1 -> two_pole_filter/1
  Mirrored Leg Length Target/2(dl_leg) -> Mux5/2
  Mirrored Leg Length Target/3(ddl_leg) -> Mux5/3
  Mirrored Leg Length Target/1(l_leg) -> Mux5/1
  Constant4/1 -> Mux6/3
  k_virtual6/1 -> Mux6/2
  Fcn2/1 -> Mux6/1
  Move Leg to Apex Target [1/0]/1 -> Detect Change/1, Switch/2
  Mux7/1 -> Demux6/1, Switch/3
  Mux9/1 -> Mux10/1
  Mux8/1 -> Mux10/2
  Mux10/1 -> Switch/1
  Torso Pitch [rad rad/s]/1 -> Selector/1, Sum1/1
  Selector/1 -> Virtual Leg Trajectory Towards Alpha Apex Target/3(theta)
  Mux5/1 -> Mux7/1
  Mux6/1 -> Mux7/2
  Virtual Leg Trajectory Towards Alpha Apex Target/6(ddphi) -> Mux8/3
  Virtual Leg Trajectory Towards Alpha Apex Target/5(dphi) -> Mux8/2
  Virtual Leg Trajectory Towards Alpha Apex Target/4(phi) -> Mux8/1
  Virtual Leg Trajectory Towards Alpha Apex Target/3(ddl_leg) -> Mux9/3
  Virtual Leg Trajectory Towards Alpha Apex Target/2(dl_leg) -> Mux9/2
  Virtual Leg Trajectory Towards Alpha Apex Target/1(l_leg) -> Mux9/1
  Detect Change/1 -> Virtual Leg Trajectory Towards Alpha Apex Target/1(start)
  Clock/1 -> Virtual Leg Trajectory Towards Alpha Apex Target/2(t_system)
  Demux4/2 -> Virtual Leg Trajectory Towards Alpha Apex Target/5(dl_measured)
  Demux4/1 -> Virtual Leg Trajectory Towards Alpha Apex Target/4(l_measured)
  Demux7/1 -> Virtual Leg Trajectory Towards Alpha Apex Target/6(phi_measured)
  Demux7/2 -> Virtual Leg Trajectory Towards Alpha Apex Target/7(dphi_measured)
  Secondary Leg Length [m m/s]/1 -> Demux4/1
  Secondary Leg Angle [rad rad/s]/1 -> Demux7/1
  Virtual Leg to Four Bar/1(back) -> Avoid Hitting Mechanical Limits/1(back_desired)
  Virtual Leg to Four Bar/2(dback) -> Avoid Hitting Mechanical Limits/2(dback_desired)
  Virtual Leg to Four Bar/3(ddback) -> Avoid Hitting Mechanical Limits/3(ddback_desired)
  Virtual Leg to Four Bar/4(front) -> Avoid Hitting Mechanical Limits/4(front_desired)
  Virtual Leg to Four Bar/5(dfront) -> Avoid Hitting Mechanical Limits/5(dfront_desired)
  Virtual Leg to Four Bar/6(ddfront) -> Avoid Hitting Mechanical Limits/6(ddfront_desired)
  Demux6/1 -> Virtual Leg to Four Bar/1(l_leg)
  Demux6/2 -> Virtual Leg to Four Bar/2(dl_leg)
  Demux6/3 -> Virtual Leg to Four Bar/3(ddl_leg)
  Demux6/4 -> Virtual Leg to Four Bar/4(phi)
  Demux6/5 -> Virtual Leg to Four Bar/5(dphi)
  Demux6/6 -> Virtual Leg to Four Bar/6(ddphi)
  Mux11/1 -> Back/Front Motor PD/5(Measured Velocity [rad/s] [back front])
  Demux2/2 -> Mux11/2
  Mux4/1 -> Back/Front Motor PD/4(Measured Position [rad] [back front])
  Mux1/1 -> Back/Front Motor PD/1(Desired Position [rad] [back front])
  Right/Left Secondary [1/0]/1 -> Back/Front Motor PD/6(Right/Left Leg [1/0])
  Demux3/2 -> Mux11/1
  Demux3/1 -> Mux4/1
  Avoid Hitting Mechanical Limits/2(front_cmd) -> Mux1/2
  Avoid Hitting Mechanical Limits/1(back_cmd) -> Mux1/1
  Demux2/1 -> Mux4/2
  Secondary Front Gear [rad rad/s]/1 -> Demux2/1
  Secondary Back Gear [rad rad/s]/1 -> Demux3/1
  Avoid Hitting Mechanical Limits/3(dback_cmd) -> Mux2/1
  Avoid Hitting Mechanical Limits/4(dfront_cmd) -> Mux2/2
  Avoid Hitting Mechanical Limits/5(ddback_cmd) -> Mux3/1
  Avoid Hitting Mechanical Limits/6(ddfront_cmd) -> Mux3/2
  Mux2/1 -> Back/Front Motor PD/2(Desired Velocity [rad/s] [back front])
  Mux3/1 -> Back/Front Motor PD/3(Desired Acceleration [rad/s^2] [back front])
  two_pole_filter/1 -> Sum1/2
  Sum1/1 -> Demux5/1
  Demux1/1 -> Mirrored Leg Length Target/1(primary_l_leg)
  Demux1/2 -> Mirrored Leg Length Target/2(primary_dl_leg)
  Primary Leg Length [m m/s]/1 -> Demux1/1

== system smm_with_grf_tilting_2d/Control/Behavior Control/Torque Distribution Left ==
  Leg Torque [Nm] : Inport
  Leg Force [N] : Inport  Port=2
  w [m] : Inport  Port=3
  Gain : Gain  Gain=0.5
  Gain1 : Gain  Gain=0.5
  Motor Torque Saturation Optimization : MATLAB Function  TreatAsAtomicUnit=on
  Product : Product  RndMeth=Zero
  Sum : Sum  Inputs=|++
  Sum1 : Sum  Inputs=+-|
  Back Torque [Nm] : Outport
  Front Torque [Nm] : Outport  Port=2
  wires:
  Gain/1 -> Motor Torque Saturation Optimization/1(x1s)
  Gain1/1 -> Motor Torque Saturation Optimization/2(x2s)
  Product/1 -> Gain1/1
  Leg Force [N]/1 -> Product/1
  Motor Torque Saturation Optimization/2(t2) -> Sum/2, Sum1/2
  w [m]/1 -> Product/2
  Motor Torque Saturation Optimization/1(t1) -> Sum1/1, Sum/1
  Sum/1 -> Front Torque [Nm]/1
  Leg Torque [Nm]/1 -> Gain/1
  Sum1/1 -> Back Torque [Nm]/1

== system smm_with_grf_tilting_2d/Control/Behavior Control/Torque Distribution Right ==
  Leg Torque [Nm] : Inport
  Leg Force [N] : Inport  Port=2
  w [m] : Inport  Port=3
  Gain : Gain  Gain=0.5
  Gain1 : Gain  Gain=0.5
  Motor Torque Saturation Optimization : MATLAB Function  TreatAsAtomicUnit=on
  Product : Product  RndMeth=Zero
  Sum : Sum  Inputs=|++
  Sum1 : Sum  Inputs=+-|
  Back Torque [Nm] : Outport
  Front Torque [Nm] : Outport  Port=2
  wires:
  Sum1/1 -> Back Torque [Nm]/1
  Leg Torque [Nm]/1 -> Gain/1
  Sum/1 -> Front Torque [Nm]/1
  Motor Torque Saturation Optimization/1(t1) -> Sum/1, Sum1/1
  w [m]/1 -> Product/2
  Motor Torque Saturation Optimization/2(t2) -> Sum1/2, Sum/2
  Leg Force [N]/1 -> Product/1
  Product/1 -> Gain1/1
  Gain1/1 -> Motor Torque Saturation Optimization/2(x2s)
  Gain/1 -> Motor Torque Saturation Optimization/1(x1s)
